simulink model "machine_frigo"  (R2021a)
settings: Solver=VariableStepAuto  StartTime=0.0  StopTime=120000  RelTol=1e-3
undefined symbols (not defined in the file): cuivre_densite, e_conduite, e_mur, H_conduite, L_conduite, P_data, R_conduite, ro_baie, ro_mur, S_haut, S_laterale, S_mur, Surface_max, Surface_min, Tcons, Text, Tmax_detendeur, Tmin_detendeur, v_baie, v_mur
libraries: fl_lib x47, nesl_utility x9
settings Model: Creator=Etudiant  LastModifiedBy=ethan
settings SolverCC: MaxConsecutiveMinStep=3  AlgebraicLoopSolver=TrustRegion
settings DebuggingCC: ParameterPrecisionLossMsg=none  SFMachineParentedDataDiag=warning

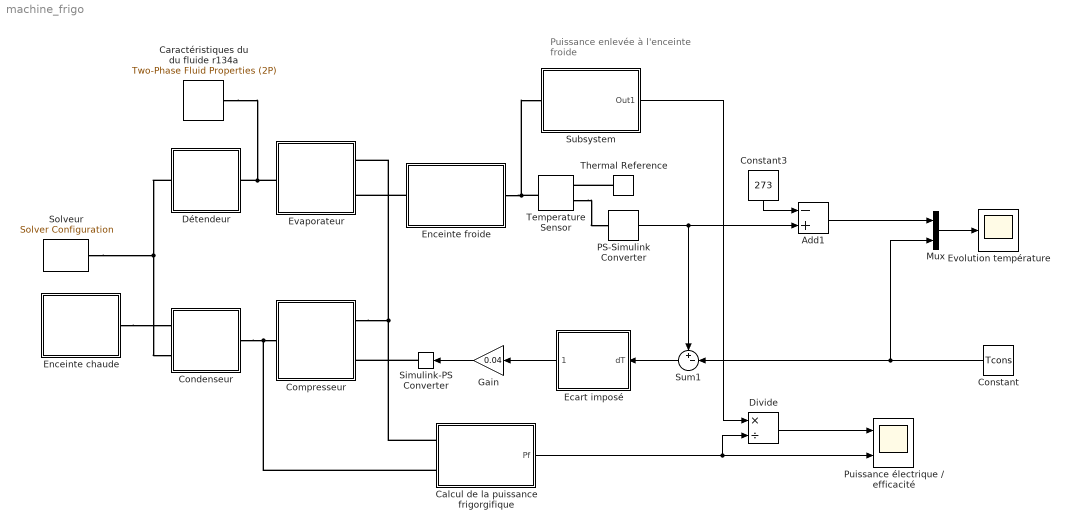
== system machine_frigo ==
  note: Puissance enlevée
      | à l'enceinte froide
  Add1 : Sum  Inputs=-+
  Calcul de la puissance frigorgifique : Subsystem
  Caractéristiques du du fluide r134a : fl_lib/Two-Phase Fluid/Utilities/Two-Phase Fluid Properties (2P)  u_min=r134aPropertyTables.u_min kJ/kg  u_max=r134aPropertyTables.u_max kJ/kg  unorm_liq=r134aPropertyTables.liquid.unorm  unorm_vap=r134aPropertyTables.vapor.unorm  p_TLU=r134aPropertyTables.p MPa  v_liq=r134aPropertyTables.liquid.v m^3/kg  v_vap=r134aPropertyTables.vapor.v m^3/kg  s_liq=r134aPropertyTables.liquid.s kJ/kg/K  s_vap=r134aPropertyTables.vapor.s kJ/kg/K  T_liq=r134aPropertyTables.liquid.T K  T_vap=r134aPropertyTables.vapor.T K  nu_liq=r134aPropertyTables.liquid.nu mm^2/s  nu_vap=r134aPropertyTables.vapor.nu mm^2/s  k_liq=r134aPropertyTables.liquid.k W/(m*K)  k_vap=r134aPropertyTables.vapor.k W/(m*K)  Pr_liq=r134aPropertyTables.liquid.Pr  Pr_vap=r134aPropertyTables.vapor.Pr  u_sat_liq=r134aPropertyTables.liquid.u_sat kJ/kg  u_sat_vap=r134aPropertyTables.vapor.u_sat kJ/kg  p_crit=r134aPropertyTables.p_crit MPa  critical_region=foundation.enum.critical_region.clip  p_crit_fraction=0.12  p_atm=0.101325 MPa  q_rev=0.01 Pa
      settings: SourceProductBaseCode=SS  InternalSimscapePortConfiguration="{\"Bottom\":[],\"Left\":[],\"Right\":[{\"id\":\"A\",\"label\":\"\",\"type\":\"foundation.two_phase_fluid.two_phase_fluid\"}],\"Top\":[]}"
  Compresseur : Subsystem
  "Condenseur " : Subsystem
  Constant : Constant  Value=Tcons
  Constant3 : Constant  Value=273
  Divide : Product  Inputs=*/
  "Détendeur " : Subsystem
  Ecart imposé : Subsystem
  Enceinte chaude : Subsystem
  "Enceinte froide " : Subsystem
  Evaporateur : Subsystem
  Evolution température : Scope
  Gain : Gain  Gain=0.04
  Mux : Mux  Inputs=2
  PS-Simulink Converter : nesl_utility/PS-Simulink Converter  PhysicalDomain=network_engine_domain  SubClassName=ps_output  LeftPortType=input  RightPortType=output  PseudoPeriodic=off  Frequencies=[]  Unit=K  AffineConversion=off
      settings: SourceProductBaseCode=PW,SS
  Puissance électrique / efficacité : Scope  NumInputPorts=2
  Simulink-PS Converter : nesl_utility/Simulink-PS Converter  PhysicalDomain=network_engine_domain  SubClassName=ps_input  LeftPortType=input  RightPortType=output  PseudoPeriodic=off  Frequencies=[]  NoiseDistribution=none  NoiseParameters=[]  Unit=1  AffineConversion=off  FilteringAndDerivatives=provide  SimscapeFilterOrder=1  InputFilterTimeConstant=0.001  UdotUserProvided=0
      settings: SourceProductBaseCode=PW,SS
  Solveur : nesl_utility/Solver Configuration  PhysicalDomain=network_engine_domain  SubClassName=solver  LeftPortType=input  RightPortType=generic  Tones=[]  Harmonics=[]  SimulateNoise=off  Profile=off  UseLocalSampling=off  EnableSwitchedLinearOptims=on  FrequencyDomain=off  UseCCode=off  RelTol=0.001  AbsTol=1e-06  MinStep=1e-09  ToWorkspace=off  RevertToSquareIcSolve=off  NumHomotopyIterations=100  PhasorMode=off  PhasorModeNumHarmonics=1  DoDC=off  ResidualTolerance=1e-9  UseLocalSolver=off  LocalSolverChoice=NE_BACKWARD_EULER_ADVANCER  LocalSolverSampleTime=1  DoFixedCost=off  MaxNonlinIter=3  MaxModeIter=2  ComputeImpulses=off  ImpulseIterations=2  LinearAlgebra=auto  EquationFormulation=NE_TIME_EF  DelaysMemoryBudget=1024  AutomaticFiltering=off  FilteringTimeConstant=0.001  PartitionStorageMethod=AS_NEEDED  PartitionMemoryBudget=1024  PartitionMethod=ROBUST
      settings: SourceProductBaseCode=PW,SS
  Subsystem : Subsystem
  Sum1 : Sum  Inputs=+-|
  Temperature Sensor : fl_lib/Thermal/Thermal Sensors/Temperature Sensor
  Thermal Reference : fl_lib/Thermal/Thermal Elements/Thermal Reference
  wires:
  Mux/1 -> Evolution température/1
  Constant3/1 -> Add1/1
  Ecart imposé/1(1) -> Gain/1
  PS-Simulink Converter/1 -> Sum1/1, Add1/2
  Constant/1 -> Mux/2, Sum1/2
  Gain/1 -> Simulink-PS Converter/1
  Sum1/1 -> Ecart imposé/1(dT)
  Add1/1 -> Mux/1
  Subsystem/1(Out1) -> Divide/1
  Calcul de la puissance frigorgifique/1(Pf) -> Divide/2, Puissance électrique / efficacité/2
  Divide/1 -> Puissance électrique / efficacité/1
  connections:
  "Enceinte froide "/LConn1 -- Evaporateur/RConn2
  Evaporateur/LConn1 -- Caractéristiques du du fluide r134a/RConn1 -- "Détendeur "/LConn1
  "Détendeur "/RConn1 -- Solveur/RConn1 -- "Condenseur "/LConn2
  "Condenseur "/RConn1 -- Calcul de la puissance frigorgifique/LConn2 -- Compresseur/RConn1
  Compresseur/LConn1 -- Calcul de la puissance frigorgifique/LConn1 -- Evaporateur/RConn1
  Thermal Reference/LConn1 -- Temperature Sensor/RConn1
  Temperature Sensor/RConn2 -- PS-Simulink Converter/LConn1
  Enceinte chaude/RConn1 -- "Condenseur "/LConn1
  Simulink-PS Converter/RConn1 -- Compresseur/LConn2
  "Enceinte froide "/RConn1 -- Temperature Sensor/LConn1 -- Subsystem/LConn1

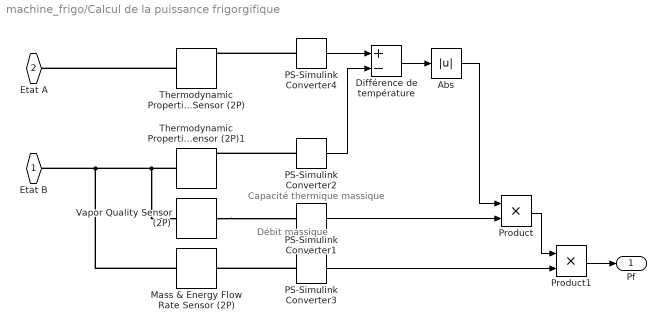
== system machine_frigo/Calcul de la puissance frigorgifique ==
  note: Débit massique
  note: Capacité thermique
      | massique
  Abs : Abs
  Différence de température : Sum  Inputs=+-
  Mass & Energy Flow Rate Sensor (2P) : fl_lib/Two-Phase Fluid/Sensors/Mass & Energy Flow Rate Sensor (2P)
      settings: SourceProductBaseCode=SS  InternalSimscapePortConfiguration="{\"Bottom\":[],\"Left\":[{\"id\":\"A\",\"label\":\"A\",\"type\":\"foundation.two_phase_fluid.two_phase_fluid\"}],\"Right\":[{\"id\":\"B\",\"label\":\"B\",\"type\":\"foundation.two_phase_fluid.two_phase_fluid\"},{\"id\":\"M\",\"label\":\"M\",\"type\":\"output\"},{\"id\":\"PHI\",\"label\":\"Phi\",\"type\":\"output\"}],\"Top\":[]}"
  PS-Simulink Converter1 : nesl_utility/PS-Simulink Converter  PhysicalDomain=network_engine_domain  SubClassName=ps_output  LeftPortType=input  RightPortType=output  PseudoPeriodic=off  Frequencies=[]  Unit=kJ/(kg*K)  AffineConversion=off
      settings: SourceProductBaseCode=PW,SS
  PS-Simulink Converter2 : nesl_utility/PS-Simulink Converter  PhysicalDomain=network_engine_domain  SubClassName=ps_output  LeftPortType=input  RightPortType=output  PseudoPeriodic=off  Frequencies=[]  Unit=K  AffineConversion=off
      settings: SourceProductBaseCode=PW,SS
  PS-Simulink Converter3 : nesl_utility/PS-Simulink Converter  PhysicalDomain=network_engine_domain  SubClassName=ps_output  LeftPortType=input  RightPortType=output  PseudoPeriodic=off  Frequencies=[]  Unit=kg/s  AffineConversion=off
      settings: SourceProductBaseCode=PW,SS
  PS-Simulink Converter4 : nesl_utility/PS-Simulink Converter  PhysicalDomain=network_engine_domain  SubClassName=ps_output  LeftPortType=input  RightPortType=output  PseudoPeriodic=off  Frequencies=[]  Unit=K  AffineConversion=off
      settings: SourceProductBaseCode=PW,SS
  Product : Product
  Product1 : Product
  Thermodynamic Properties Sensor (2P) : fl_lib/Two-Phase Fluid/Sensors/Thermodynamic Properties Sensor (2P)
      settings: SourceProductBaseCode=SS  InternalSimscapePortConfiguration="{\"Bottom\":[],\"Left\":[{\"id\":\"A\",\"label\":\"A\",\"type\":\"foundation.two_phase_fluid.two_phase_fluid\"}],\"Right\":[{\"id\":\"T\",\"label\":\"T\",\"type\":\"output\"},{\"id\":\"H\",\"label\":\"h\",\"type\":\"output\"},{\"id\":\"V\",\"label\":\"v\",\"type\":\"output\"},{\"id\":\"S\",\"label\":\"s\",\"type\":\"output\"}],\"Top\":[]}"
  Thermodynamic Properties Sensor (2P)1 : fl_lib/Two-Phase Fluid/Sensors/Thermodynamic Properties Sensor (2P)
      settings: SourceProductBaseCode=SS  InternalSimscapePortConfiguration="{\"Bottom\":[],\"Left\":[{\"id\":\"A\",\"label\":\"A\",\"type\":\"foundation.two_phase_fluid.two_phase_fluid\"}],\"Right\":[{\"id\":\"T\",\"label\":\"T\",\"type\":\"output\"},{\"id\":\"H\",\"label\":\"h\",\"type\":\"output\"},{\"id\":\"V\",\"label\":\"v\",\"type\":\"output\"},{\"id\":\"S\",\"label\":\"s\",\"type\":\"output\"}],\"Top\":[]}"
  Vapor Quality Sensor (2P) : fl_lib/Two-Phase Fluid/Sensors/Vapor Quality Sensor (2P)  vapor_fraction_spec=foundation.enum.vapor_fraction_spec.quality
      settings: SourceProductBaseCode=SS  InternalSimscapePortConfiguration="{\"Bottom\":[],\"Left\":[{\"id\":\"A\",\"label\":\"A\",\"type\":\"foundation.two_phase_fluid.two_phase_fluid\"}],\"Right\":[{\"id\":\"X\",\"label\":\"X\",\"type\":\"output\"}],\"Top\":[]}"
  Etat B : PMIOPort  Side=Left
  Etat A : PMIOPort  Port=2  Side=Left
  Pf : Outport  Unit=kW
  wires:
  Product1/1 -> Pf/1
  PS-Simulink Converter4/1 -> Différence de température/1
  Différence de température/1 -> Abs/1
  PS-Simulink Converter2/1 -> Différence de température/2
  Product/1 -> Product1/1
  PS-Simulink Converter1/1 -> Product/2
  Abs/1 -> Product/1
  PS-Simulink Converter3/1 -> Product1/2
  connections:
  Thermodynamic Properties Sensor (2P)1/LConn1 -- Vapor Quality Sensor (2P)/LConn1 -- Mass & Energy Flow Rate Sensor (2P)/LConn1 -- Etat B/RConn1
  Thermodynamic Properties Sensor (2P)/LConn1 -- Etat A/RConn1
  PS-Simulink Converter4/LConn1 -- Thermodynamic Properties Sensor (2P)/RConn1
  PS-Simulink Converter2/LConn1 -- Thermodynamic Properties Sensor (2P)1/RConn1
  Vapor Quality Sensor (2P)/RConn1 -- PS-Simulink Converter1/LConn1
  PS-Simulink Converter3/LConn1 -- Mass & Energy Flow Rate Sensor (2P)/RConn2

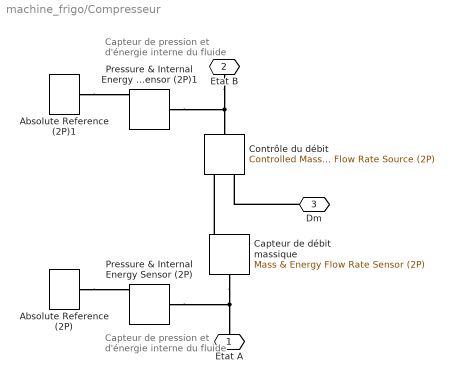
== system machine_frigo/Compresseur ==
  note: Capteur de pression
      | et d'énergie interne
      | du fluide
  note: Capteur de pression
      | et d'énergie interne
      | du fluide
  Absolute Reference (2P) : fl_lib/Two-Phase Fluid/Elements/Absolute Reference (2P)
      settings: SourceProductBaseCode=SS
  Absolute Reference (2P)1 : fl_lib/Two-Phase Fluid/Elements/Absolute Reference (2P)
      settings: SourceProductBaseCode=SS
  Capteur de débit massique : fl_lib/Two-Phase Fluid/Sensors/Mass & Energy Flow Rate Sensor (2P)
      settings: SourceProductBaseCode=SS  InternalSimscapePortConfiguration="{\"Bottom\":[],\"Left\":[{\"id\":\"A\",\"label\":\"A\",\"type\":\"foundation.two_phase_fluid.two_phase_fluid\"}],\"Right\":[{\"id\":\"B\",\"label\":\"B\",\"type\":\"foundation.two_phase_fluid.two_phase_fluid\"},{\"id\":\"M\",\"label\":\"M\",\"type\":\"output\"},{\"id\":\"PHI\",\"label\":\"Phi\",\"type\":\"output\"}],\"Top\":[]}"
  Contrôle du débit : fl_lib/Two-Phase Fluid/Sources/Controlled Mass Flow Rate Source (2P)  power_spec=foundation.enum.power_spec.isentropic  area_A=pi*R_conduite^2 m^2  area_B=pi*R_conduite^2 m^2
      settings: SourceProductBaseCode=SS  InternalSimscapePortConfiguration="{\"Bottom\":[],\"Left\":[{\"id\":\"A\",\"label\":\"A\",\"type\":\"foundation.two_phase_fluid.two_phase_fluid\"},{\"id\":\"M\",\"label\":\"M\",\"type\":\"input\"}],\"Right\":[{\"id\":\"B\",\"label\":\"B\",\"type\":\"foundation.two_phase_fluid.two_phase_fluid\"}],\"Top\":[]}"
  Pressure & Internal Energy Sensor (2P) : fl_lib/Two-Phase Fluid/Sensors/Pressure & Internal Energy Sensor (2P)
      settings: SourceProductBaseCode=SS  InternalSimscapePortConfiguration="{\"Bottom\":[],\"Left\":[{\"id\":\"A\",\"label\":\"A\",\"type\":\"foundation.two_phase_fluid.two_phase_fluid\"}],\"Right\":[{\"id\":\"B\",\"label\":\"B\",\"type\":\"foundation.two_phase_fluid.two_phase_fluid\"},{\"id\":\"P\",\"label\":\"P\",\"type\":\"output\"},{\"id\":\"U\",\"label\":\"U\",\"type\":\"output\"}],\"Top\":[]}"
  Pressure & Internal Energy Sensor (2P)1 : fl_lib/Two-Phase Fluid/Sensors/Pressure & Internal Energy Sensor (2P)
      settings: SourceProductBaseCode=SS  InternalSimscapePortConfiguration="{\"Bottom\":[],\"Left\":[{\"id\":\"A\",\"label\":\"A\",\"type\":\"foundation.two_phase_fluid.two_phase_fluid\"}],\"Right\":[{\"id\":\"B\",\"label\":\"B\",\"type\":\"foundation.two_phase_fluid.two_phase_fluid\"},{\"id\":\"P\",\"label\":\"P\",\"type\":\"output\"},{\"id\":\"U\",\"label\":\"U\",\"type\":\"output\"}],\"Top\":[]}"
  Etat A : PMIOPort  Side=Left
  Etat B : PMIOPort  Port=2  Side=Right
  Dm : PMIOPort  Port=3  Side=Left
  connections:
  Capteur de débit massique/LConn1 -- Pressure & Internal Energy Sensor (2P)/LConn1 -- Etat A/RConn1
  Etat B/RConn1 -- Pressure & Internal Energy Sensor (2P)1/LConn1 -- Contrôle du débit/RConn1
  Capteur de débit massique/RConn1 -- Contrôle du débit/LConn1
  Absolute Reference (2P)/LConn1 -- Pressure & Internal Energy Sensor (2P)/RConn1
  Absolute Reference (2P)1/LConn1 -- Pressure & Internal Energy Sensor (2P)1/RConn1
  Dm/RConn1 -- Contrôle du débit/LConn2

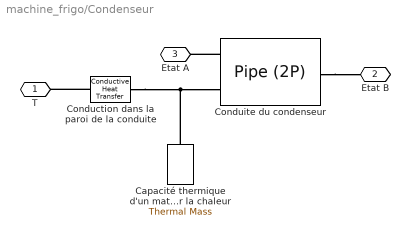
== system machine_frigo/Condenseur  ==
  Capacité thermique d'un matériau à conserver la chaleur : fl_lib/Thermal/Thermal Elements/Thermal Mass  mass=pi*2*R_conduite*H_conduite*e_conduite*cuivre_densite kg  sp_heat=Cuivre_chaleur J/kg/K  T_specify=on  T_priority=High  T=Text K  T_nominal_specify=off  T_nominal_unit=K  T_nominal_value=1  Q_specify=off  Q_priority=None  Q=0 W  Q_nominal_specify=off  Q_nominal_unit=W  Q_nominal_value=1
  Conduction dans la paroi de la conduite : fl_lib/Thermal/Thermal Elements/Conductive Heat Transfer  area=pi*2*R_conduite*H_conduite m^2  thickness=e_conduite m  th_cond=lambda_cuivre W/(m*K)  T_specify=off  T_priority=None  T=0 K  T_nominal_specify=off  T_nominal_unit=K  T_nominal_value=1  Q_specify=off  Q_priority=None  Q=0 W  Q_nominal_specify=off  Q_nominal_unit=W  Q_nominal_value=1
  "Conduite du condenseur " : fl_lib/Two-Phase Fluid/Elements/Pipe (2P)  length=H_conduite m  area=pi*R_conduite^2 m^2  Dh=R_conduite*2 m  length_add=0.1*H_conduite mm  roughness=1.5e-5 m  Re_lam=2e+3  Re_tur=4e+3  shape_factor=64  Nu_lam=3.66  inertia=simscape.enum.onoff.off  energy_spec=foundation.enum.energy_spec.quality  p_init=Pinit bar  T_init=293.15 K  x_init=Qinit_vap  alpha_init=0.5  h_init=1500 kJ/kg  u_init=1500 kJ/kg  mdot_init=0 kg/s  time_constant=0.1 s
      settings: SourceProductBaseCode=SS  InternalSimscapePortConfiguration="{\"Bottom\":[],\"Left\":[{\"id\":\"A\",\"label\":\"A\",\"type\":\"foundation.two_phase_fluid.two_phase_fluid\"},{\"id\":\"H\",\"label\":\"H\",\"type\":\"foundation.thermal.thermal\"}],\"Right\":[{\"id\":\"B\",\"label\":\"B\",\"type\":\"foundation.two_phase_fluid.two_phase_fluid\"}],\"Top\":[]}"
  T : PMIOPort  Side=Left
  Etat B : PMIOPort  Port=2  Side=Left
  Etat A : PMIOPort  Port=3  Side=Right
  connections:
  Capacité thermique d'un matériau à conserver la chaleur/LConn1 -- "Conduite du condenseur "/LConn2 -- Conduction dans la paroi de la conduite/LConn1
  Conduction dans la paroi de la conduite/RConn1 -- T/RConn1
  "Conduite du condenseur "/RConn1 -- Etat B/RConn1
  "Conduite du condenseur "/LConn1 -- Etat A/RConn1

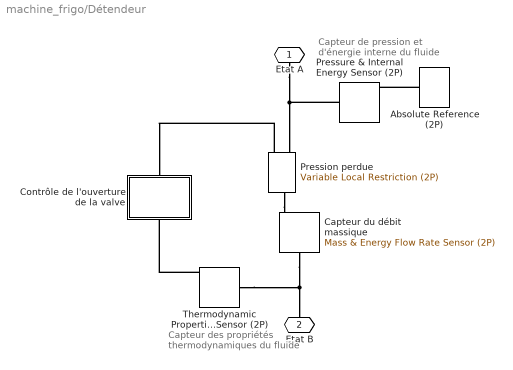
== system machine_frigo/Détendeur  ==
  note: Capteur des propriétés
      | thermodynamiques du
      | fluide
  note: Capteur de pression
      | et d'énergie interne
      | du fluide
  Absolute Reference (2P) : fl_lib/Two-Phase Fluid/Elements/Absolute Reference (2P)
      settings: SourceProductBaseCode=SS
  "Capteur du débit massique " : fl_lib/Two-Phase Fluid/Sensors/Mass & Energy Flow Rate Sensor (2P)
      settings: SourceProductBaseCode=SS  InternalSimscapePortConfiguration="{\"Bottom\":[],\"Left\":[{\"id\":\"A\",\"label\":\"A\",\"type\":\"foundation.two_phase_fluid.two_phase_fluid\"}],\"Right\":[{\"id\":\"B\",\"label\":\"B\",\"type\":\"foundation.two_phase_fluid.two_phase_fluid\"},{\"id\":\"M\",\"label\":\"M\",\"type\":\"output\"},{\"id\":\"PHI\",\"label\":\"Phi\",\"type\":\"output\"}],\"Top\":[]}"
  Contrôle de l'ouverture de la valve : Subsystem
  Pression perdue : fl_lib/Two-Phase Fluid/Elements/Variable Local Restriction (2P)  min_area=Surface_min mm^2  max_area=Surface_max mm^2  area=pi*R_conduite^2 m^2  Cd=0.7  B_lam=0.999
      settings: SourceProductBaseCode=SS  InternalSimscapePortConfiguration="{\"Bottom\":[],\"Left\":[{\"id\":\"A\",\"label\":\"A\",\"type\":\"foundation.two_phase_fluid.two_phase_fluid\"},{\"id\":\"area_in\",\"label\":\"AR\",\"type\":\"input\"}],\"Right\":[{\"id\":\"B\",\"label\":\"B\",\"type\":\"foundation.two_phase_fluid.two_phase_fluid\"}],\"Top\":[]}"
  Pressure & Internal Energy Sensor (2P) : fl_lib/Two-Phase Fluid/Sensors/Pressure & Internal Energy Sensor (2P)
      settings: SourceProductBaseCode=SS  InternalSimscapePortConfiguration="{\"Bottom\":[],\"Left\":[{\"id\":\"A\",\"label\":\"A\",\"type\":\"foundation.two_phase_fluid.two_phase_fluid\"}],\"Right\":[{\"id\":\"B\",\"label\":\"B\",\"type\":\"foundation.two_phase_fluid.two_phase_fluid\"},{\"id\":\"P\",\"label\":\"P\",\"type\":\"output\"},{\"id\":\"U\",\"label\":\"U\",\"type\":\"output\"}],\"Top\":[]}"
  Thermodynamic Properties Sensor (2P) : fl_lib/Two-Phase Fluid/Sensors/Thermodynamic Properties Sensor (2P)
      settings: SourceProductBaseCode=SS  InternalSimscapePortConfiguration="{\"Bottom\":[],\"Left\":[{\"id\":\"A\",\"label\":\"A\",\"type\":\"foundation.two_phase_fluid.two_phase_fluid\"}],\"Right\":[{\"id\":\"T\",\"label\":\"T\",\"type\":\"output\"},{\"id\":\"H\",\"label\":\"h\",\"type\":\"output\"},{\"id\":\"V\",\"label\":\"v\",\"type\":\"output\"},{\"id\":\"S\",\"label\":\"s\",\"type\":\"output\"}],\"Top\":[]}"
  Etat A : PMIOPort  Side=Left
  Etat B : PMIOPort  Port=2  Side=Right
  connections:
  Pressure & Internal Energy Sensor (2P)/LConn1 -- Etat A/RConn1 -- Pression perdue/LConn1
  "Capteur du débit massique "/LConn1 -- Thermodynamic Properties Sensor (2P)/LConn1 -- Etat B/RConn1
  Pression perdue/RConn1 -- "Capteur du débit massique "/RConn1
  Pression perdue/LConn2 -- Contrôle de l'ouverture de la valve/LConn1
  Absolute Reference (2P)/LConn1 -- Pressure & Internal Energy Sensor (2P)/RConn1
  Thermodynamic Properties Sensor (2P)/RConn1 -- Contrôle de l'ouverture de la valve/RConn1

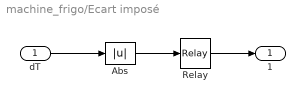
== system machine_frigo/Ecart imposé ==
  dT : Inport
  Abs : Abs
  Relay : Relay  OnSwitchValue=2.1  OffSwitchValue=2
  1 : Outport  VectorParamsAs1DForOutWhenUnconnected=off
  wires:
  dT/1 -> Abs/1
  Relay/1 -> 1/1
  Abs/1 -> Relay/1

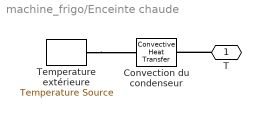
== system machine_frigo/Enceinte chaude ==
  Convection du condenseur : fl_lib/Thermal/Thermal Elements/Convective Heat Transfer  area=S_fin m^2  heat_tr_coeff=h_fin W/(m^2 * K)  T_specify=off  T_priority=None  T=0 K  T_nominal_specify=off  T_nominal_unit=K  T_nominal_value=1  Q_specify=off  Q_priority=None  Q=0 W  Q_nominal_specify=off  Q_nominal_unit=W  Q_nominal_value=1
  Temperature extérieure : fl_lib/Thermal/Thermal Sources/Temperature Source  temperature=Text K
  T : PMIOPort  Side=Right
  connections:
  Temperature extérieure/LConn1 -- Convection du condenseur/LConn1
  T/RConn1 -- Convection du condenseur/RConn1

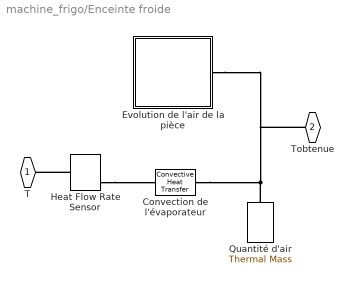
== system machine_frigo/Enceinte froide  ==
  Convection de l'évaporateur : fl_lib/Thermal/Thermal Elements/Convective Heat Transfer  area=Sint m^2  heat_tr_coeff=h_air W/(m^2 * K)  T_specify=off  T_priority=None  T=0 K  T_nominal_specify=off  T_nominal_unit=K  T_nominal_value=1  Q_specify=off  Q_priority=None  Q=0 W  Q_nominal_specify=off  Q_nominal_unit=W  Q_nominal_value=1
  "Evolution de l'air de la pièce " : Subsystem
  Heat Flow Rate Sensor : fl_lib/Thermal/Thermal Sensors/Heat Flow Rate Sensor
      settings: SourceProductBaseCode=SS
  Quantité d'air : fl_lib/Thermal/Thermal Elements/Thermal Mass  mass=1000*25 kg  sp_heat=1012 J/kg/K  T_specify=on  T_priority=High  T=Tcons K  T_nominal_specify=off  T_nominal_unit=K  T_nominal_value=1  Q_specify=off  Q_priority=None  Q=0 W  Q_nominal_specify=off  Q_nominal_unit=W  Q_nominal_value=1
  T : PMIOPort  Side=Left
  Tobtenue : PMIOPort  Port=2  Side=Right
  connections:
  Quantité d'air/LConn1 -- Tobtenue/RConn1 -- "Evolution de l'air de la pièce "/LConn1 -- Convection de l'évaporateur/RConn1
  Heat Flow Rate Sensor/RConn2 -- Convection de l'évaporateur/LConn1
  Heat Flow Rate Sensor/LConn1 -- T/RConn1

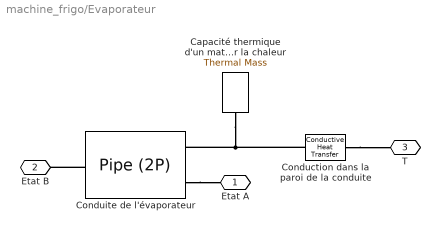
== system machine_frigo/Evaporateur ==
  Capacité thermique d'un matériau à conserver la chaleur : fl_lib/Thermal/Thermal Elements/Thermal Mass  mass=pi*2*R_conduite*L_conduite*e_conduite*cuivre_densite kg  sp_heat=Cuivre_chaleur J/kg/K  T_specify=on  T_priority=High  T=Tcons K  T_nominal_specify=off  T_nominal_unit=K  T_nominal_value=1  Q_specify=off  Q_priority=None  Q=0 W  Q_nominal_specify=off  Q_nominal_unit=W  Q_nominal_value=1
  Conduction dans la paroi de la conduite : fl_lib/Thermal/Thermal Elements/Conductive Heat Transfer  area=pi*2*R_conduite*L_conduite m^2  thickness=e_conduite m  th_cond=lambda_cuivre W/(m*K)  T_specify=off  T_priority=None  T=0 K  T_nominal_specify=off  T_nominal_unit=K  T_nominal_value=1  Q_specify=off  Q_priority=None  Q=0 W  Q_nominal_specify=off  Q_nominal_unit=W  Q_nominal_value=1
  Conduite de l'évaporateur : fl_lib/Two-Phase Fluid/Elements/Pipe (2P)  length=L_conduite m  area=pi*R_conduite^2 m^2  Dh=2*R_conduite m  length_add=0.1*L_conduite mm  roughness=1.5e-5 m  Re_lam=2e+3  Re_tur=4e+3  shape_factor=64  Nu_lam=3.66  inertia=simscape.enum.onoff.off  energy_spec=foundation.enum.energy_spec.quality  p_init=Pinit bar  T_init=293.15 K  x_init=Qinit_vap  alpha_init=0.5  h_init=1500 kJ/kg  u_init=1500 kJ/kg  mdot_init=0 kg/s  time_constant=0.1 s
      settings: SourceProductBaseCode=SS  InternalSimscapePortConfiguration="{\"Bottom\":[],\"Left\":[{\"id\":\"A\",\"label\":\"A\",\"type\":\"foundation.two_phase_fluid.two_phase_fluid\"},{\"id\":\"H\",\"label\":\"H\",\"type\":\"foundation.thermal.thermal\"}],\"Right\":[{\"id\":\"B\",\"label\":\"B\",\"type\":\"foundation.two_phase_fluid.two_phase_fluid\"}],\"Top\":[]}"
  Etat A : PMIOPort  Side=Left
  Etat B : PMIOPort  Port=2  Side=Right
  T : PMIOPort  Port=3  Side=Right
  connections:
  Capacité thermique d'un matériau à conserver la chaleur/LConn1 -- Conduite de l'évaporateur/LConn2 -- Conduction dans la paroi de la conduite/LConn1
  Conduction dans la paroi de la conduite/RConn1 -- T/RConn1
  Conduite de l'évaporateur/LConn1 -- Etat A/RConn1
  Conduite de l'évaporateur/RConn1 -- Etat B/RConn1

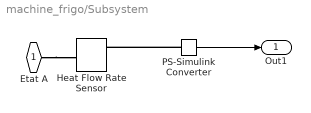
== system machine_frigo/Subsystem ==
  Heat Flow Rate Sensor : fl_lib/Thermal/Thermal Sensors/Heat Flow Rate Sensor
      settings: SourceProductBaseCode=SS
  PS-Simulink Converter : nesl_utility/PS-Simulink Converter  PhysicalDomain=network_engine_domain  SubClassName=ps_output  LeftPortType=input  RightPortType=output  PseudoPeriodic=off  Frequencies=[]  Unit=inherit  AffineConversion=off
      settings: SourceProductBaseCode=PW,SS
  Etat A : PMIOPort  Side=Left
  Out1 : Outport
  wires:
  PS-Simulink Converter/1 -> Out1/1
  connections:
  PS-Simulink Converter/LConn1 -- Heat Flow Rate Sensor/RConn1
  Etat A/RConn1 -- Heat Flow Rate Sensor/LConn1

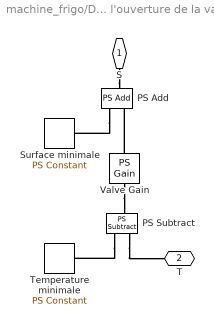
== system machine_frigo/Détendeur /Contrôle de l'ouverture de la valve ==
  PS Add : fl_lib/Physical Signals/Functions/PS Add
  PS Subtract : fl_lib/Physical Signals/Functions/PS Subtract
  Surface minimale : fl_lib/Physical Signals/Sources/PS Constant  constant=Surface_min mm^2
  Temperature minimale : fl_lib/Physical Signals/Sources/PS Constant  constant=Tmin_detendeur K
  Valve Gain : fl_lib/Physical Signals/Functions/PS Gain  gain=(Surface_max - Surface_min)/(Tmax_detendeur - Tmin_detendeur) mm^2/K
  S : PMIOPort  Side=Left
  T : PMIOPort  Port=2  Side=Right
  connections:
  PS Subtract/LConn1 -- T/RConn1
  PS Add/LConn1 -- Surface minimale/RConn1
  PS Subtract/LConn2 -- Temperature minimale/RConn1
  Valve Gain/LConn1 -- PS Subtract/RConn1
  Valve Gain/RConn1 -- PS Add/LConn2
  S/RConn1 -- PS Add/RConn1

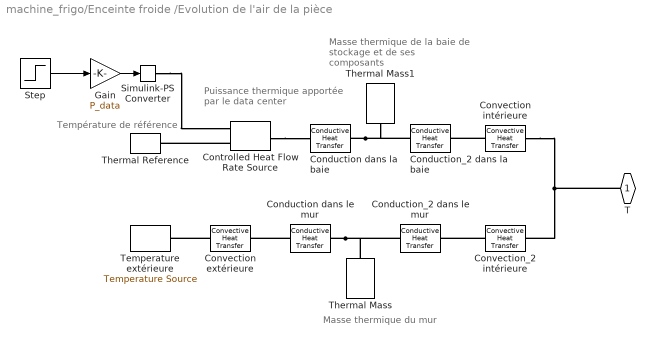
== system machine_frigo/Enceinte froide /Evolution de l'air de la pièce  ==
  note: Température
      | de référence
  note: Masse thermique
      |         du mur
  note: Puissance thermique
      | apportée par le data
      | 	     center
  note: Masse thermique de la
      | baie de stockage et de
      |      ses composants
  Conduction dans la baie : fl_lib/Thermal/Thermal Elements/Conductive Heat Transfer  area=4*S_laterale+S_haut m^2  thickness=0.05 m  th_cond=lambda_baie W/(m*K)  T_specify=off  T_priority=None  T=0 K  T_nominal_specify=off  T_nominal_unit=K  T_nominal_value=1  Q_specify=off  Q_priority=None  Q=0 W  Q_nominal_specify=off  Q_nominal_unit=W  Q_nominal_value=1
  Conduction dans le mur : fl_lib/Thermal/Thermal Elements/Conductive Heat Transfer  area=4*S_mur m^2  thickness=e_mur/2 m  th_cond=lambda_mur W/(m*K)  T_specify=off  T_priority=None  T=0 K  T_nominal_specify=off  T_nominal_unit=K  T_nominal_value=1  Q_specify=off  Q_priority=None  Q=0 W  Q_nominal_specify=off  Q_nominal_unit=W  Q_nominal_value=1
  Conduction_2 dans la baie : fl_lib/Thermal/Thermal Elements/Conductive Heat Transfer  area=4*S_laterale+S_haut m^2  thickness=0.05 m  th_cond=lambda_baie W/(m*K)  T_specify=off  T_priority=None  T=0 K  T_nominal_specify=off  T_nominal_unit=K  T_nominal_value=1  Q_specify=off  Q_priority=None  Q=0 W  Q_nominal_specify=off  Q_nominal_unit=W  Q_nominal_value=1
  Conduction_2 dans le mur : fl_lib/Thermal/Thermal Elements/Conductive Heat Transfer  area=4*S_mur m^2  thickness=e_mur/2 m  th_cond=lambda_mur W/(m*K)  T_specify=off  T_priority=None  T=0 K  T_nominal_specify=off  T_nominal_unit=K  T_nominal_value=1  Q_specify=off  Q_priority=None  Q=0 W  Q_nominal_specify=off  Q_nominal_unit=W  Q_nominal_value=1
  Controlled Heat Flow Rate Source : fl_lib/Thermal/Thermal Sources/Controlled Heat Flow Rate Source
  Convection extérieure : fl_lib/Thermal/Thermal Elements/Convective Heat Transfer  area=4*S_mur m^2  heat_tr_coeff=h_air W/(m^2 * K)  T_specify=off  T_priority=None  T=0 K  T_nominal_specify=off  T_nominal_unit=K  T_nominal_value=1  Q_specify=off  Q_priority=None  Q=0 W  Q_nominal_specify=off  Q_nominal_unit=W  Q_nominal_value=1
      settings: LogSimulationData=on
  Convection intérieure : fl_lib/Thermal/Thermal Elements/Convective Heat Transfer  area=4*S_laterale+S_haut m^2  heat_tr_coeff=h_air W/(m^2 * K)  T_specify=off  T_priority=None  T=0 K  T_nominal_specify=off  T_nominal_unit=K  T_nominal_value=1  Q_specify=off  Q_priority=None  Q=0 W  Q_nominal_specify=off  Q_nominal_unit=W  Q_nominal_value=1
      settings: LogSimulationData=on
  Convection_2 intérieure : fl_lib/Thermal/Thermal Elements/Convective Heat Transfer  area=4*S_mur m^2  heat_tr_coeff=h_air W/(m^2 * K)  T_specify=off  T_priority=None  T=0 K  T_nominal_specify=off  T_nominal_unit=K  T_nominal_value=1  Q_specify=off  Q_priority=None  Q=0 W  Q_nominal_specify=off  Q_nominal_unit=W  Q_nominal_value=1
      settings: LogSimulationData=on
  Gain : Gain  Gain=P_data
  Simulink-PS Converter : nesl_utility/Simulink-PS Converter  PhysicalDomain=network_engine_domain  SubClassName=ps_input  LeftPortType=input  RightPortType=output  PseudoPeriodic=off  Frequencies=[]  NoiseDistribution=none  NoiseParameters=[]  Unit=1  AffineConversion=off  FilteringAndDerivatives=provide  SimscapeFilterOrder=1  InputFilterTimeConstant=0.001  UdotUserProvided=0
      settings: SourceProductBaseCode=PW,SS
  Step : Step  SampleTime=0
  Temperature extérieure : fl_lib/Thermal/Thermal Sources/Temperature Source  temperature=Text K
  Thermal Mass : fl_lib/Thermal/Thermal Elements/Thermal Mass  mass=ro_mur*v_mur kg  sp_heat=Cp_mur J/kg/K  T_specify=on  T_priority=High  T=Tcons K  T_nominal_specify=off  T_nominal_unit=K  T_nominal_value=1  Q_specify=off  Q_priority=None  Q=0 W  Q_nominal_specify=off  Q_nominal_unit=W  Q_nominal_value=1
  Thermal Mass1 : fl_lib/Thermal/Thermal Elements/Thermal Mass  mass=ro_baie*v_baie kg  sp_heat=Cp_baie J/kg/K  T_specify=on  T_priority=High  T=Tcons K  T_nominal_specify=off  T_nominal_unit=K  T_nominal_value=1  Q_specify=off  Q_priority=None  Q=0 W  Q_nominal_specify=off  Q_nominal_unit=W  Q_nominal_value=1
  Thermal Reference : fl_lib/Thermal/Thermal Elements/Thermal Reference
  T : PMIOPort  Side=Left
  wires:
  Step/1 -> Gain/1
  Gain/1 -> Simulink-PS Converter/1
  connections:
  Conduction dans la baie/RConn1 -- Conduction_2 dans la baie/LConn1 -- Thermal Mass1/LConn1
  Convection intérieure/RConn1 -- T/RConn1 -- Convection_2 intérieure/RConn1
  Controlled Heat Flow Rate Source/RConn2 -- Thermal Reference/LConn1
  Conduction dans le mur/RConn1 -- Thermal Mass/LConn1 -- Conduction_2 dans le mur/LConn1
  Convection_2 intérieure/LConn1 -- Conduction_2 dans le mur/RConn1
  Convection intérieure/LConn1 -- Conduction_2 dans la baie/RConn1
  Controlled Heat Flow Rate Source/LConn1 -- Conduction dans la baie/LConn1
  Convection extérieure/LConn1 -- Temperature extérieure/LConn1
  Conduction dans le mur/LConn1 -- Convection extérieure/RConn1
  Simulink-PS Converter/RConn1 -- Controlled Heat Flow Rate Source/RConn1
